simulink model "data_trajectory_true"  (R2016b)
settings: Solver=ode1  StartTime=0.0  StopTime=50  FixedStep=0.01  RelTol=1e-3
undefined symbols (not defined in the file or in its folder): deg, rad, s
libraries: simulink x6, aerolibconvert2 x2, aerolib6dof2 x1, dspsrcs4 x1
settings Model: Creator=Utente  LastModifiedBy=Utente

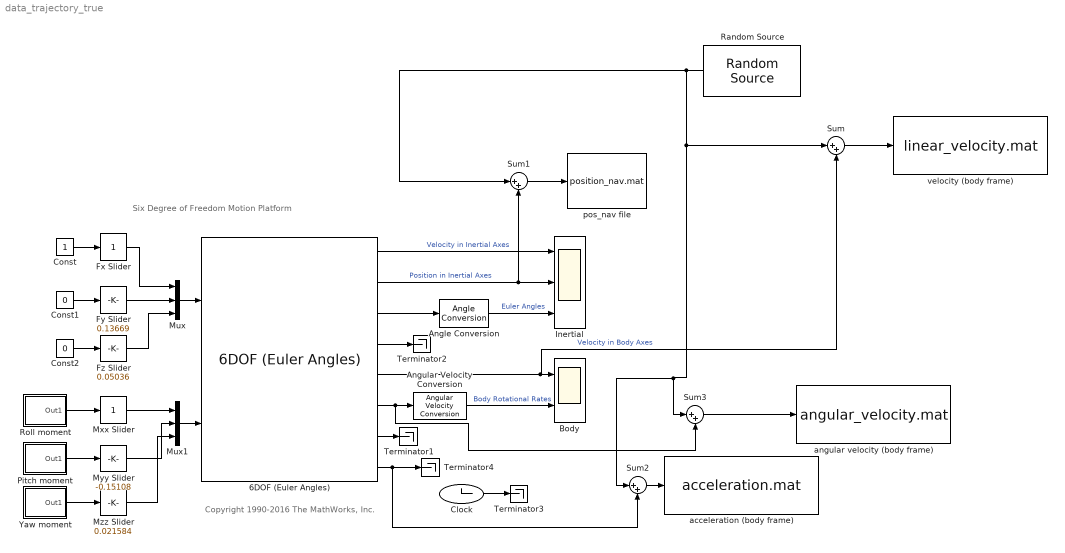
== system data_trajectory_true ==
  note: Six Degree of Freedom Motion Platform
  note: Copyright 1990-2016 The MathWorks, Inc.
  6DOF (Euler Angles) : aerolib6dof2/6DOF (Euler Angles)  units=Metric (MKS)  mtype=Fixed  rep=Euler Angles  xme_0=[0 0 0]  Vm_0=[0 0 0]  eul_0=[0 0 0]  pm_0=[0 0 0]  mass_0=1.0  mass_e=0.5  mass_f=2.0  inertia=eye(3)  inertia_e=eye(3)  inertia_f=2*eye(3)  k_quat=1.0  vre_flag=on
  Angle Conversion : aerolibconvert2/Angle Conversion  IU=rad  OU=deg
  Angular Velocity Conversion : aerolibconvert2/Angular Velocity Conversion  IU=rad/s  OU=deg/s
  Body : Scope  NumInputPorts=2
  Clock : Clock
      settings: Decimation=100
  Const : Constant
  Const1 : Constant  Value=0
  Const2 : Constant  Value=0
  Fx Slider : simulink/Math Operations/Slider Gain  low=-1  gain=1  high=1
  Fy Slider : simulink/Math Operations/Slider Gain  low=-1  gain=0.13669  high=1
  Fz Slider : simulink/Math Operations/Slider Gain  low=-1  gain=0.05036  high=1
  Inertial : Scope  NumInputPorts=3
  Mux : Mux  Inputs=3
  Mux1 : Mux  Inputs=3
  Mxx Slider : simulink/Math Operations/Slider Gain  low=0  gain=1  high=1
  Myy Slider : simulink/Math Operations/Slider Gain  low=-1  gain=-0.15108  high=1
  Mzz Slider : simulink/Math Operations/Slider Gain  low=-1  gain=0.021584  high=3
  Pitch moment : Subsystem  mask(timed input){t=[0 3 3 4 4 5 5  7.5 7.5 8.5 8.5 9.5 9.5 10], u=[0 0  1 1 -1 -1.005 0 0 -1 -1 1 1 0 0]*3.138/2}
      mask prompts: t "time values:"; u "input values"
      mask Display: plot(t,u)
  Random Source : dspsrcs4/Random Source  SrcType=Gaussian  NormMethod=Ziggurat  CltLength=12  MinVal=0  MaxVal=1  MeanVal=[0; 0; 0]  VarVal=[0.05; 0.05; 0.05]  RepMode=Not repeatable  rawSeed=1  IsInherit=off  SampMode=Discrete  SampTime=-1  SampFrame=1  DataType=Double  OutComplex=Real  OutputFrames=off
  Roll moment : Subsystem  mask(timed input){t=[0 1 1 2 2  10], u=[1 1 -1 -.998  0 0]*3.144/2}
      mask prompts: t "time values:"; u "input values"
      mask Display: plot(t,u)
  Sum{,1..3} (4 alike) : Sum  Inputs=|++
  Terminator{1..4} (4 alike) : Terminator
  Yaw moment : Subsystem  mask(timed input){t=[0 6 6 7 7 8 8 10], u=[0 0  -1 -1 1 1 0 0]*3.1/2}
      mask prompts: t "time values:"; u "input values"
      mask Display: plot(t,u)
  acceleration (body frame) : ToFile  Filename=acceleration.mat  MatrixName=acc  SaveFormat=Timeseries
  angular velocity (body frame) : ToFile  Filename=angular_velocity.mat  MatrixName=av  SaveFormat=Timeseries
  pos_nav file : ToFile  Filename=position_nav.mat  MatrixName=pos_nav  SaveFormat=Timeseries
  velocity (body frame) : ToFile  Filename=linear_velocity.mat  MatrixName=lv  SaveFormat=Timeseries
  wires:
  Yaw moment/1(Out1) -> Mzz Slider/1
  Pitch moment/1(Out1) -> Myy Slider/1
  Roll moment/1(Out1) -> Mxx Slider/1
  Const2/1 -> Fz Slider/1
  Const1/1 -> Fy Slider/1
  Const/1 -> Fx Slider/1
  Clock/1 -> Terminator3/1
  Mux1/1 -> 6DOF (Euler Angles)/2
  Mzz Slider/1 -> Mux1/3
  Myy Slider/1 -> Mux1/2
  Mxx Slider/1 -> Mux1/1
  Mux/1 -> 6DOF (Euler Angles)/1
  Fy Slider/1 -> Mux/2
  Fz Slider/1 -> Mux/3
  Fx Slider/1 -> Mux/1
  6DOF (Euler Angles)/4 -> Terminator2/1
  6DOF (Euler Angles)/7 -> Terminator1/1
  6DOF (Euler Angles)/3 -> Angle Conversion/1
  6DOF (Euler Angles)/5 -> Sum/2, Body/1  "Velocity in Body Axes"
  6DOF (Euler Angles)/1 -> Inertial/1  "Velocity in Inertial Axes"
  6DOF (Euler Angles)/2 -> Inertial/2, Sum1/2  "Position in Inertial Axes"
  Angle Conversion/1 -> Inertial/3  "Euler Angles"
  6DOF (Euler Angles)/6 -> Sum3/2, Angular Velocity Conversion/1
  Angular Velocity Conversion/1 -> Body/2  "Body Rotational Rates"
  6DOF (Euler Angles)/8 -> Sum2/2, Terminator4/1
  Random Source/1 -> Sum/1, Sum2/1, Sum3/1, Sum1/1
  Sum/1 -> velocity (body frame)/1
  Sum1/1 -> pos_nav file/1
  Sum2/1 -> acceleration (body frame)/1
  Sum3/1 -> angular velocity (body frame)/1

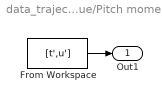
== system data_trajectory_true/Pitch moment ==
  From Workspace : FromWorkspace  VariableName=[t',u']  SampleTime=0
  Out1 : Outport
  wires:
  From Workspace/1 -> Out1/1

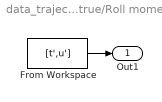
== system data_trajectory_true/Roll moment ==
  From Workspace : FromWorkspace  VariableName=[t',u']  SampleTime=0
  Out1 : Outport
  wires:
  From Workspace/1 -> Out1/1

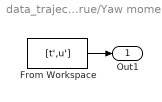
== system data_trajectory_true/Yaw moment ==
  From Workspace : FromWorkspace  VariableName=[t',u']  SampleTime=0
  Out1 : Outport
  wires:
  From Workspace/1 -> Out1/1
